simulink model "CruiseControl_TestGen_DisengageWithBrake_Seq_"  (R2018b)
settings: Solver=FixedStepDiscrete  StartTime=0.0  StopTime=2  FixedStep=0.1  RelTol=1e-3  EnableMultiTasking=on
settings Model: DataDictionary=CruiseControl_Req_dd.sldd  Creator=colosky  LastModifiedBy=colosky
settings DataIOCC: LimitDataPoints=on  SaveFormat=Array  SaveOutput=off  SaveTime=off
settings OptimizationCC: DefaultParameterBehavior=Inlined  InlineInvariantSignals=on  ExpressionDepthLimit=2147483647  InitFltsAndDblsToZero=on  NoFixptDivByZeroProtection=on  LifeSpan=inf
settings DebuggingCC: SignalInfNanChecking=warning  SaveWithParameterizedLinksMsg=none  UnderspecifiedInitializationDetection=Classic  MergeDetectMultiDrivingBlocksExec=none  SolverPrmCheckMsg=warning  FcnCallInpInsideContextMsg=warning  UniqueDataStoreMsg=warning  AllowSymbolicDim=off  StateNameClashWarn=warning  StrictBusMsg=ErrorOnBusTreatedAsVector  SFUnexpectedBacktrackingDiag=warning  SFNoUnconditionalDefaultTransitionDiag=warning  SFExecutionAtInitializationDiag=none
settings HardwareCC: ProdBitPerPointer=32  ProdBitPerSizeT=32  ProdBitPerPtrDiffT=32  ProdLargestAtomicFloat=None  ProdEndianess=Unspecified  ProdWordSize=32  ProdHWDeviceType=32-bit Generic
settings ModelReferenceCC: ModelReferenceNumInstancesAllowed=Single  PropagateSignalLabelsOutOfModel=off
settings SFSimCC: SimUseLocalCustomCode=off  SimParseCustomCode=off  MATLABDynamicMemAlloc=off
settings RTWCC: SystemTargetFile=ert.tlc  TemplateMakefile=ert_default_tmf  GenerateReport=on  RTWUseLocalCustomCode=off  IncludeHyperlinkInReport=on  LaunchReport=on  PortableWordSizes=on  GenerateTraceInfo=on  GenerateTraceReport=on  GenerateTraceReportSl=on  GenerateTraceReportSf=on  GenerateTraceReportEml=on
settings CodeAppCC: IgnoreCustomStorageClasses=off  CustomSymbolStrGlobalVar=$N$M  StateflowObjectComments=on
settings ERTTargetCC: MultiwordLength=2048  GenerateSampleERTMain=on  InlinedParameterPlacement=NonHierarchical  ERTCustomFileTemplate=example_file_process.tlc  ConvertIfToSwitch=off  SuppressUnreachableDefaultCases=off
settings ConfigComp: CovScope=ReferencedModels  CovIncludeTopModel=off  CovMetricSettings=dcme  CovExternalEMLEnable=off  CovSFcnEnable=off  DVMode=DesignErrorDetection  DVMaxProcessTime=3000  DVDisplayUnsatisfiableObjectives=on  DVAutomaticStubbing=off  DVMakeOutputFilesUnique=off  DVModelCoverageObjectives=None  DVMaxTestCaseSteps=500  DVTestSuiteOptimization=IndividualObjectives  DVAssertions=EnableAll  DVProofAssumptions=EnableAll  DVCoverageDataFile=CruiseControlCovManual.cvt  DVDetectDeadLogic=on  DVDetectActiveLogic=on  DVDetectIntegerOverflow=off  DVMaxViolationSteps=50  DVSaveExpectedOutput=on  DVHarnessModelFileName=$ModelName$_harness_SLDV  DVReportIncludeGraphics=on  PSAutoStubLUT=off

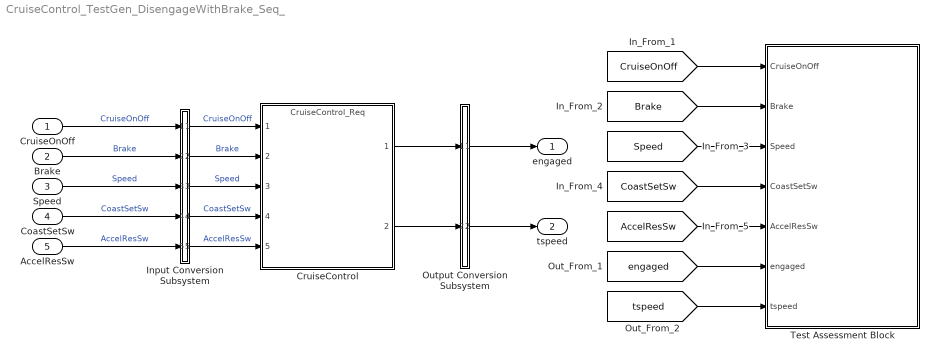
== system CruiseControl_TestGen_DisengageWithBrake_Seq_ ==
  CruiseOnOff : Inport  OutDataTypeStr=boolean  PortDimensions=[1]  SampleTime=0.1
  Brake : Inport  Port=2  OutDataTypeStr=boolean  PortDimensions=[1]  SampleTime=0.1
  Speed : Inport  Port=3  OutDataTypeStr=uint8  PortDimensions=[1]  SampleTime=0.1
  CoastSetSw : Inport  Port=4  OutDataTypeStr=boolean  PortDimensions=[1]  SampleTime=0.1
  AccelResSw : Inport  Port=5  OutDataTypeStr=boolean  PortDimensions=[1]  SampleTime=0.1
  CruiseControl : ModelReference  ModelNameDialog=CruiseControl_Req.slx  SimulationMode=Normal  ModelReferenceVersion=1.465
  Input Conversion Subsystem : Subsystem  Tag=__SLT_ICS__  Description=|
      | Signal spec.
      | and routing
      settings: AttributesFormatString=%<Description>
  Output Conversion Subsystem : Subsystem  Tag=__SLT_OCS__  Description=|
      | Signal spec.
      | and routing
      settings: AttributesFormatString=%<Description>
  Test Assessment Block : Test Sequence  Tag=__SLT_ASMT__  TreatAsAtomicUnit=on
  engaged : Outport  OutDataTypeStr=boolean  PortDimensions=[1]
  tspeed : Outport  Port=2  OutDataTypeStr=uint8  PortDimensions=[1]
  wires:
  [CruiseOnOff] -> Test Assessment Block/1(CruiseOnOff)
  [Brake] -> Test Assessment Block/2(Brake)
  [Speed] -> Test Assessment Block/3(Speed)
  [CoastSetSw] -> Test Assessment Block/4(CoastSetSw)
  [AccelResSw] -> Test Assessment Block/5(AccelResSw)
  [engaged] -> Test Assessment Block/6(engaged)
  [tspeed] -> Test Assessment Block/7(tspeed)
  CruiseOnOff/1 -> Input Conversion Subsystem/1(Inport_1)  "CruiseOnOff"
  Brake/1 -> Input Conversion Subsystem/2(Inport_2)  "Brake"
  Speed/1 -> Input Conversion Subsystem/3(Inport_3)  "Speed"
  CoastSetSw/1 -> Input Conversion Subsystem/4(Inport_4)  "CoastSetSw"
  AccelResSw/1 -> Input Conversion Subsystem/5(Inport_5)  "AccelResSw"
  Output Conversion Subsystem/1(Outport_1) -> engaged/1
  Output Conversion Subsystem/2(Outport_2) -> tspeed/1
  Input Conversion Subsystem/1(Outport_1) -> CruiseControl/1  "CruiseOnOff"
  Input Conversion Subsystem/2(Outport_2) -> CruiseControl/2  "Brake"
  Input Conversion Subsystem/3(Outport_3) -> CruiseControl/3  "Speed"
  Input Conversion Subsystem/4(Outport_4) -> CruiseControl/4  "CoastSetSw"
  Input Conversion Subsystem/5(Outport_5) -> CruiseControl/5  "AccelResSw"
  CruiseControl/1 -> Output Conversion Subsystem/1(Inport_1)
  CruiseControl/2 -> Output Conversion Subsystem/2(Inport_2)

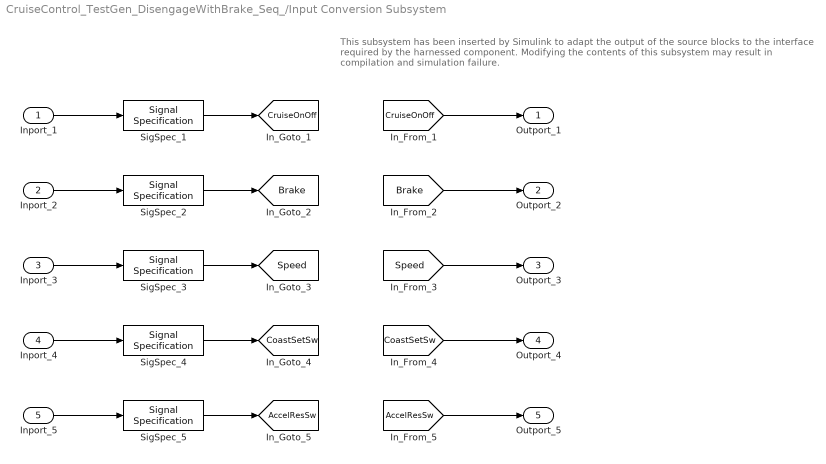
== system CruiseControl_TestGen_DisengageWithBrake_Seq_/Input Conversion Subsystem ==
  note: This subsystem has been inserted by Simulink to adapt the output of the source blocks to the interface required by the harnessed component.
      |  Modifying the contents of this subsystem may result in compilation and simulation failure.
  Inport_1 : Inport
  Inport_2 : Inport  Port=2
  Inport_3 : Inport  Port=3
  Inport_4 : Inport  Port=4
  Inport_5 : Inport  Port=5
  SigSpec_{1..2,4..5} (4 alike) : SignalSpecification  OutDataTypeStr=boolean  Dimensions=[1]  SampleTime=0.1
  SigSpec_3 : SignalSpecification  OutDataTypeStr=uint8  Dimensions=[1]  SampleTime=0.1
  Outport_1 : Outport
  Outport_2 : Outport  Port=2
  Outport_3 : Outport  Port=3
  Outport_4 : Outport  Port=4
  Outport_5 : Outport  Port=5
  tag scope: AccelResSw=global, Brake=global, CoastSetSw=global, CruiseOnOff=global, Speed=global
  wires:
  [CruiseOnOff] -> Outport_1/1
  SigSpec_1/1 -> [CruiseOnOff]
  Inport_1/1 -> SigSpec_1/1
  [Brake] -> Outport_2/1
  SigSpec_2/1 -> [Brake]
  Inport_2/1 -> SigSpec_2/1
  [Speed] -> Outport_3/1
  SigSpec_3/1 -> [Speed]
  Inport_3/1 -> SigSpec_3/1
  [CoastSetSw] -> Outport_4/1
  SigSpec_4/1 -> [CoastSetSw]
  Inport_4/1 -> SigSpec_4/1
  [AccelResSw] -> Outport_5/1
  SigSpec_5/1 -> [AccelResSw]
  Inport_5/1 -> SigSpec_5/1

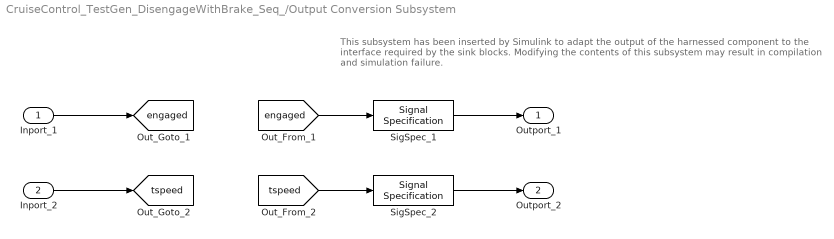
== system CruiseControl_TestGen_DisengageWithBrake_Seq_/Output Conversion Subsystem ==
  note: This subsystem has been inserted by Simulink to adapt the output of the harnessed component to the interface required by the sink blocks.
      |  Modifying the contents of this subsystem may result in compilation and simulation failure.
  Inport_1 : Inport
  Inport_2 : Inport  Port=2
  SigSpec_1 : SignalSpecification  OutDataTypeStr=boolean  Dimensions=[1]  SampleTime=0.1
  SigSpec_2 : SignalSpecification  OutDataTypeStr=uint8  Dimensions=[1]  SampleTime=0.1
  Outport_1 : Outport
  Outport_2 : Outport  Port=2
  tag scope: engaged=global, tspeed=global
  wires:
  Inport_1/1 -> [engaged]
  [engaged] -> SigSpec_1/1
  SigSpec_1/1 -> Outport_1/1
  Inport_2/1 -> [tspeed]
  [tspeed] -> SigSpec_2/1
  SigSpec_2/1 -> Outport_2/1

== stateflow chart CruiseControl_TestGen_DisengageWithBrake_Seq_/Test Assessment Block ==
  settings: stateMachineType=SIMPLIFIED_MACHINE
  state Init
    BrakeLast = Brake;
    engagedLast = engaged;
  state TestGen
    % Disengage With Brake
    sldv.condition(Speed>=20 && Speed<=90);
    TO_DisengageWithBrake = Brake && ~BrakeLast && engagedLast;
    sldv.test(TO_DisengageWithBrake);
    if TO_DisengageWithBrake
    verify(~engaged, 'DisengageWithBrake:verify', ...
    'DisengageWithBrake fails');
    end
    BrakeLast = Brake;
    engagedLast = engaged;
  (default) -> Init
  Init -> TestGen
  data: CruiseOnOff input boolean size=[1]; Brake input boolean size=[1]; Speed input uint8 size=[1]; CoastSetSw input boolean size=[1]; AccelResSw input boolean size=[1]; engaged input boolean size=[1]; tspeed input uint8 size=[1]; BrakeLast local; engagedLast local; TO_DisengageWithBrake local boolean
